simulink library "hvs_mapBased_chy_std"  (R2016a)
settings: Solver=ode45  StartTime=0.0  StopTime=10.0  RelTol=1e-3
undefined symbols (not defined in the file): sMP
libraries: chy_framelib x1
settings Model: Creator=LAUEREL  LastModifiedBy=KNWINDE
settings DataIOCC: LimitDataPoints=on  SaveFormat=Array
settings OptimizationCC: ExpressionDepthLimit=2147483647
settings DebuggingCC: UnderspecifiedInitializationDetection=Classic  MergeDetectMultiDrivingBlocksExec=none  SolverPrmCheckMsg=warning  StateNameClashWarn=warning
settings HardwareCC: ProdBitPerPointer=32  ProdLargestAtomicFloat=None  ProdIntDivRoundTo=Undefined  ProdEndianess=Unspecified  ProdWordSize=32  ProdHWDeviceType=32-bit Generic
settings ModelReferenceCC: PropagateSignalLabelsOutOfModel=off
settings ConfigComp: CovModelRefEnable=Off

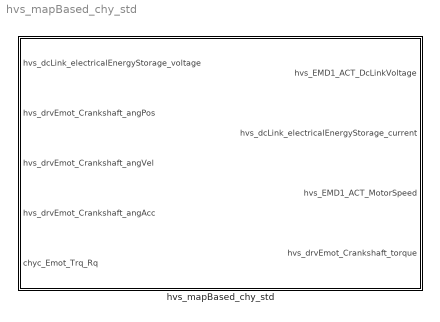
== system hvs_mapBased_chy_std ==
  hvs_mapBased_chy_std : Subsystem  mask{emot_nTab_1stD=sMP.phys.hvs.emot_nTab_1stD, emot_trqTab_2ndD=sMP.phys.hvs.emot_trqTab_2ndD, emot_vltTab_3rdD=sMP.phys.hvs.emot_vltTab_3rdD, emot_Ri_Inv=sMP.phys.hvs.emot_Ri_Inv, emot_inv_pwrLoss=sMP.phys.hvs.emot_inv_pwrLoss, emot_mot_pwrLoss=sMP.phys.hvs.emot_mot_pwrLoss, emot_trqMaxRow=sMP.phys.hvs.emot_trqMaxRow, emot_trqMinRow=sMP.phys.hvs.emot_trqMinRow, emot_dtrqEmotPtv=sMP.phys.hvs.emot_dtrqEmotPtv, emot_dtrqEmotNeg=sMP.phys.hvs.emot_dtrqEmotNeg, aux_power_flag=sMP.phys.hvs.aux_power_flag, SIGVAL_STATUS_ERROR=sMP.phys.hvs.SIGVAL_STATUS_ERROR, CONST_POWER_ERR_MODE=sMP.phys.hvs.CONST_POWER_ERR_MODE, CANOE_PANEL_ON=sMP.phys.hvs.CANOE_PANEL_ON, InvStEnable=sMP.phys.hvs.InvStEnable, InvStError=sMP.phys.hvs.InvStError, InvStReady=sMP.phys.hvs.InvStReady, InvStInit=sMP.phys.hvs.InvStInit, emot_Rth_stator_oil=sMP.phys.hvs.emot_Rth_stator_oil, emot_Cth_stator=sMP.phys.hvs.emot_Cth_stator, emot_Rth_stator_rotor=sMP.phys.hvs.emot_Rth_stator_rotor, emot_Cth_rotor=sMP.phys.hvs.emot_Cth_rotor, emot_Rth_rotor_oil=sMP.phys.hvs.emot_Rth_rotor_oil, emot_Tstator_init=sMP.phys.hvs.emot_Tstator_init, emot_Trotor_init=sMP.phys.hvs.emot_Trotor_init, inv_Cth_IGBT=sMP.phys.hvs.inv_Cth_IGBT, inv_Cth_diode=sMP.phys.hvs.inv_Cth_diode, inv_Rth_IGBT=sMP.phys.hvs.inv_Rth_IGBT, inv_R_th_Diode=sMP.phys.hvs.inv_R_th_Diode, inv_Rth_PS_cooling_plate=sMP.phys.hvs.inv_Rth_PS_cooling_plate, inv_Cth_cooling_plate=sMP.phys.hvs.inv_Cth_cooling_plate, inv_Rth_cooling_plate_coolant=sMP.phys.hvs.inv_Rth_cooling_plate_coolant, inv_n_IGBT_per_Switch=sMP.phys.hvs.inv_n_IGBT_per_Switch, inv_Tpowerstack_init=sMP.phys.hvs.inv_Tpowerstack_init, inv_Tplate_init=sMP.phys.hvs.inv_Tplate_init, inv_nTab_1stD=sMP.phys.hvs.inv_nTab_1stD, inv_trqTab_2ndD=sMP.phys.hvs.inv_trqTab_2ndD, inv_vltTab_3rdD=sMP.phys.hvs.inv_vltTab_3rdD}

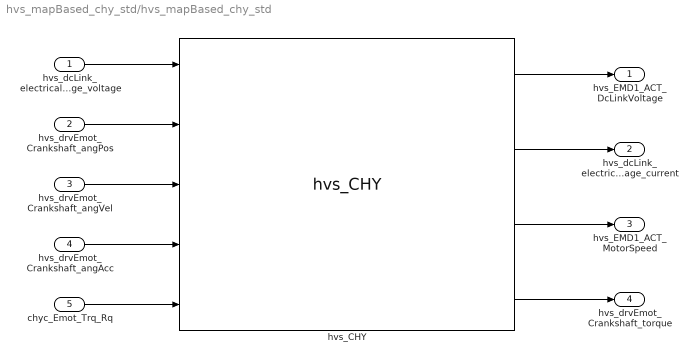
== system hvs_mapBased_chy_std/hvs_mapBased_chy_std ==
  hvs_dcLink_electricalEnergyStorage_voltage : Inport
  hvs_drvEmot_Crankshaft_angPos : Inport  Port=2
  hvs_drvEmot_Crankshaft_angVel : Inport  Port=3
  hvs_drvEmot_Crankshaft_angAcc : Inport  Port=4
  chyc_Emot_Trq_Rq : Inport  Port=5
  hvs_CHY : chy_framelib/hvs_CHY
  hvs_EMD1_ACT_DcLinkVoltage : Outport
  hvs_dcLink_electricalEnergyStorage_current : Outport  Port=2
  hvs_EMD1_ACT_MotorSpeed : Outport  Port=3
  hvs_drvEmot_Crankshaft_torque : Outport  Port=4
  wires:
  hvs_drvEmot_Crankshaft_angVel/1 -> hvs_CHY/3
  hvs_drvEmot_Crankshaft_angAcc/1 -> hvs_CHY/4
  chyc_Emot_Trq_Rq/1 -> hvs_CHY/5
  hvs_dcLink_electricalEnergyStorage_voltage/1 -> hvs_CHY/1
  hvs_drvEmot_Crankshaft_angPos/1 -> hvs_CHY/2
  hvs_CHY/1 -> hvs_EMD1_ACT_DcLinkVoltage/1
  hvs_CHY/2 -> hvs_dcLink_electricalEnergyStorage_current/1
  hvs_CHY/3 -> hvs_EMD1_ACT_MotorSpeed/1
  hvs_CHY/4 -> hvs_drvEmot_Crankshaft_torque/1
